simulink model "SModel_VolturnUS"  (R2024b)
settings: Solver=ode4  StartTime=0  StopTime=1000  FixedStep=0.01  MaxStep=0.01  RelTol=1e-3
values from neighbouring files (symbols this model uses):
  simu = simulationClass()    [wecSimInputFile.m]
undefined symbols (not defined in the file or in its folder): body, constraint, mooring, X, Y, Z
libraries: nesl_utility x18, sm_lib x11, WECSim_Lib_Body_Elements x2, WECSim_Lib_Constraints x1, WECSim_Lib_Frames x1, WECSim_Lib_Moorings x1, MOST_Lib x1
settings Model: Creator=massi  LastModifiedBy=akeeste
settings SolverCC: ZeroCrossControl=DisableAll  AlgebraicLoopSolver=TrustRegion  AutoInsertRateTranBlk=on
settings DataIOCC: ReturnWorkspaceOutputs=off
settings OptimizationCC: ReuseModelBlockBuffer=off  SimCompilerOptimization=on
settings DebuggingCC: UnconnectedInputMsg=warning  UnconnectedOutputMsg=warning  UnconnectedLineMsg=warning
settings ModelReferenceCC: EnableRefExpFcnMdlSchedulingChecks=on
settings RTWCC: GPUComputeCapability=3.5
settings ExplorerConfigSet: InternalSimMechanicsExplorerSettings="<ExplorerConfiguration><canonicalview>default</canonicalview><AnimationSetting><BasePlaybackSpeed>1.0</BasePlaybackSpeed><PlaybackSpeedFactor>64.0</PlaybackSpeedFactor></AnimationSetting><TilePanel><TileInfo><Tiles Columns=\"1\" Count=\"1\" Rows=\"1\"><Column Weight=\"1\"/><Row Weight=\"1\"/><Tile Height=\"1\" Width=\"1\" X=\"0\" Y=\"0\"/></Tiles></TileInfo><SceneInfo><SceneViewer><BGColor><R>0.800000011920928955</R><G>1</G><B>1</B></BGColor><Camera><DoPerspective>off</DoPerspective><Position><X>3.83527572012098972e-06</X><Y>-435.132249170182718</Y><Z>-23.2456610583153065</Z></Position><Center><X>3.83527572012098972e-06</X><Y>-1.30964724540660882e-05</Y><Z>-23.2456610583153065</Z></Center><Up><X>0</X><Y>-0</Y><Z>1</Z></Up><ViewLimDist>1</ViewLimDist><YLim>286.086963500976594</YLim><XLim>444.426516742997762</XLim></Camera></SceneViewer></SceneInfo></TilePanel><MechEditorPanel><Cameras/><GfxPanelCameraMap/><VideoCreator><PlaybackSpeedRatio>1.0</PlaybackSpeedRatio><FrameRate>30</FrameRate><VideoFormat>Motion JPEG AVI</VideoFormat><FrameSize>auto</FrameSize></VideoCreator></MechEditorPanel></ExplorerConfiguration>"

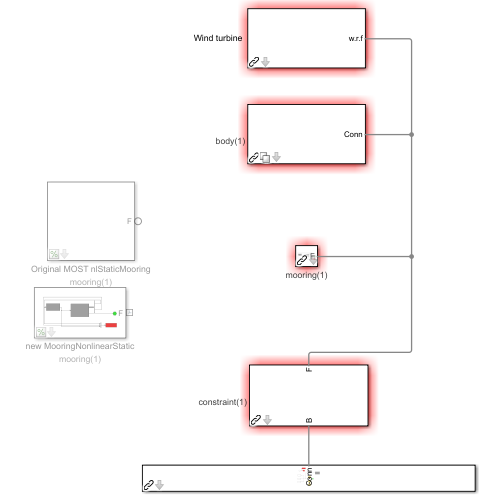
[thumbnail: Simulink's stored preview of the top-level diagram]
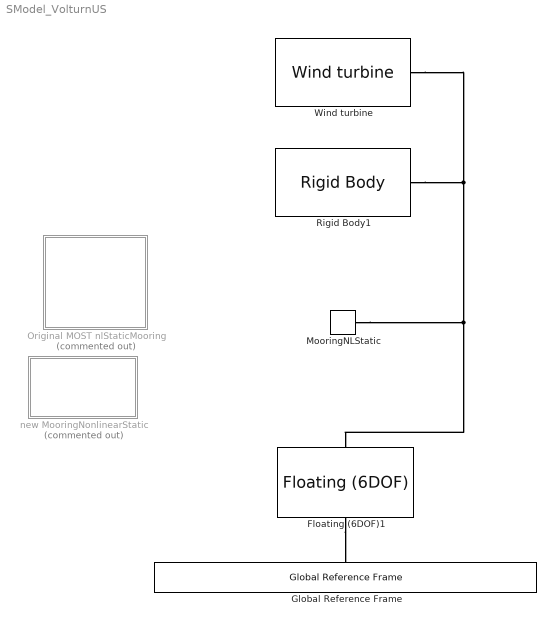
== system SModel_VolturnUS ==
  Floating (6DOF)1 : WECSim_Lib_Constraints/Floating (6DOF)  constraint=constraint(1)
      settings: AttributesFormatString=%<constraint>
  Global Reference Frame : WECSim_Lib_Frames/Global Reference Frame  waves=waves  simu=simu
  MooringNLStatic : WECSim_Lib_Moorings/MooringNLStatic  mooring=mooring(1)  nonlinearStaticData=mooring.nonlinearStaticData
      settings: AttributesFormatString=%<mooring>
  Original MOST nlStaticMooring : Subsystem  Commented=on  mask{mooring=mooring(1), Data_moor=mooring(1).nonlinearStaticData}
      mask prompts: mooring "Mooring Name:"; Data_moor "Mooring Data"
      mask init:
      | if exist('mooring','var')
      |     % toWorkSpace: outputs
      |     h=[gcb '/To Workspace'];
      |     responseName=['mooring' num2str(mooring.number) '_out'];
      |     set_param(h,'VariableName',responseName);
      | end
      settings: AttributesFormatString=%<mooring>
  Rigid Body1 : WECSim_Lib_Body_Elements/Rigid Body  body=body(1)
  Wind turbine : MOST_Lib/Wind turbine  VariantControl=sv_1_IEA15MW  windTurbine=windTurbine  BEMstruct=windTurbine.BEMstruct
      settings: SourceProductName=MOST
  new MooringNonlinearStatic : Subsystem  Commented=on  mask(Mooring Matrix){mooring=mooring(1), nonlinearStaticData=mooring.nonlinearStaticData}
      mask prompts: mooring "Mooring Name:"; nonlinearStaticData "Mooring Data"
      mask help:
      | A mooring body that applies stiffness, damping and pretensions forces to the follower. The response of the mooring body is relative to the global reference frame.
      |
      | The variable name input below must be 'mooring(i)' where i=1,2,...
      | mooring(i) must be defined in the input file with the following fields:
      |
      |     .name (required)
      |             String.
      |             Mooring name. Must comply with Matlab's variable naming rules.
      |     .location (optional)
      |             3x1 vector [x y z] in meters.
      |             Mooring location. Default = [0 0 0]
      |     .initial (optional)
      |             Struct
      |             Contains the initial position, angle and axis of the mooring body.
      |     .initial.displacement (optional)
      |             3x1 vector [x y z] in meters.
      |             Initial linear displacement from the ref position. Default = [0 0 0]
      |             This can can be set directly or with the setInitDisp() method.
      |     .initial.axis (optional)
      |             3x1 vector [x y z]
      |             Initial angular displacement axis. Default = [0 1 0]
      |             This can can be set directly or with the setInitDisp() method.
      |     .initial.angle (optional)
      |             Float.
      |             Initial angular displacement angle about axis in radians. Default = [0 0 0]
      |             This can can be set directly or with the setInitDisp() method.
      |     .matrix (optional)
      |             Struct
      |             Contains the stiffness matrix, damping matrix and pretension of the mooring body.
      |     .matrix.stiffness (optional)
      |             6x6 vector.
      |             Mooring linear spring stiffness. Default = zeros(6)
      |     .matrix.damping (optional)
      |             6x6 vector.
      |             Mooring linear damping coefficient. Default = zeros(6)
      |     .matrix.preTension (optional)
      |             6x1 vector.
      |             Mooring preTension force. Default = [0 0 0 0 0 0]
      mask init:
      | if exist('mooring','var')
      |     % toWorkSpace: outputs
      |     h=[gcb '/To Workspace'];
      |     responseName=['mooring' num2str(mooring.number) '_out'];
      |     set_param(h,'VariableName',responseName);
      | end
      settings: AttributesFormatString=%<mooring>
      mask Help:
      | A mooring body that applies stiffness, damping and pretensions forces to the follower. The response of the mooring body is relative to the global reference frame.
      | 
      | The variable name input below must be 'mooring(i)' where i=1,2,...
      | mooring(i) must be defined in the input file with the following fields:
      | 
      |     .name (required)
      |             String.
      |             Mooring name. Must comply with Matlab's variable naming rules.
      |     .location (optional)
      |             3x1 vector [x y z] in meters.
      |             Mooring location. Default = [0 0 0]
      |     .initial (optional)
      |             Struct
      |             Contains the initial position, angle and axis of the mooring body.
      |     .initial.displacement (optional)
      |             3x1 vector [x y z] in meters.
      |             Initial linear displacement from the ref position. Default = [0 0 0]
      |             This can can be set directly or with the setInitDisp() method.
      |     .initial.axis (optional)
      |             3x1 vector [x y z]
      |             Initial angular displacement axis. Default = [0 1 0]
      |             This can can be set directly or with the setInitDisp() method.
      |     .initial.angle (optional)
      |             Float.
      |             Initial angular displacement angle about axis in radians. Default = [0 0 0]
      |             This can can be set directly or with the setInitDisp() method.
      |     .matrix (optional)
      |             Struct
      |             Contains the stiffness matrix, damping matrix and pretension of the mooring body.
      |     .matrix.stiffness (optional)
      |             6x6 vector.
      |             Mooring linear spring stiffness. Default = zeros(6)
      |     .matrix.damping (optional)
      |             6x6 vector.
      |             Mooring linear damping coefficient. Default = zeros(6)
      |     .matrix.preTension (optional)
      |             6x1 vector.
      |             Mooring preTension force. Default = [0 0 0 0 0 0]
  connections:
  Rigid Body1/RConn1 -- Wind turbine/RConn1 -- MooringNLStatic/LConn1 -- Floating (6DOF)1/RConn1
  Floating (6DOF)1/LConn1 -- Global Reference Frame/RConn1

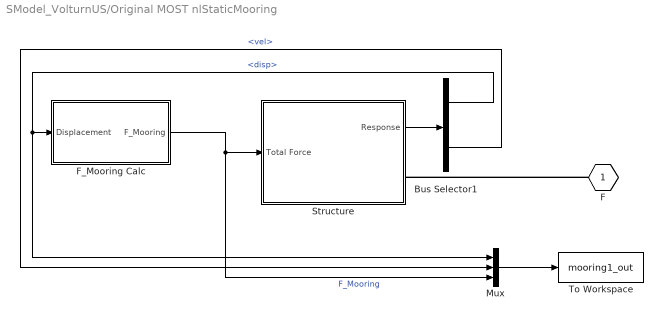
== system SModel_VolturnUS/Original MOST nlStaticMooring ==
  Bus Selector1 : BusSelector  OutputSignals=disp,vel
  F_Mooring Calc : Subsystem
  Mux : Mux  Inputs=3
  Structure : Subsystem
  To Workspace : ToWorkspace  VariableName=mooring1_out  SaveFormat=Structure With Time  SampleTime=simu.dtOut
  F : PMIOPort  Side=Left
  wires:
  Mux/1 -> To Workspace/1
  Bus Selector1/2 -> Mux/2  "<vel>"
  Bus Selector1/1 -> Mux/1, F_Mooring Calc/1(Displacement)  "<disp>"
  F_Mooring Calc/1(F_Mooring) -> Mux/3, Structure/1(Total Force)  "F_Mooring"
  Structure/1(Response) -> Bus Selector1/1
  connections:
  F/RConn1 -- Structure/RConn1

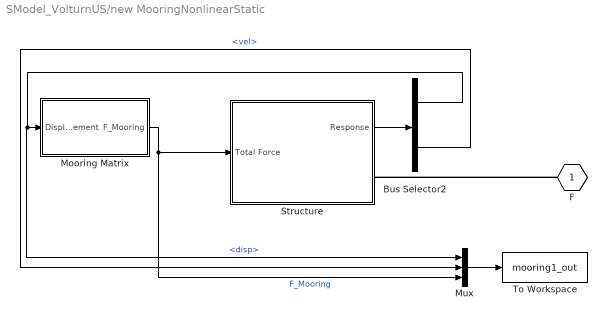
== system SModel_VolturnUS/new MooringNonlinearStatic ==
  Bus Selector2 : BusSelector  OutputSignals=disp,vel
  Mooring Matrix : Subsystem  VariantControl=sv_mooringMatrix
  Mux : Mux  Inputs=3
  Structure : Subsystem
  To Workspace : ToWorkspace  VariableName=mooring1_out  SaveFormat=Structure With Time  SampleTime=simu.dtOut
  F : PMIOPort  Side=Left
  wires:
  Mux/1 -> To Workspace/1
  Bus Selector2/2 -> Mux/2  "<vel>"
  Bus Selector2/1 -> Mooring Matrix/1(Displacement), Mux/1  "<disp>"
  Mooring Matrix/1(F_Mooring) -> Structure/1(Total Force), Mux/3  "F_Mooring"
  Structure/1(Response) -> Bus Selector2/1
  connections:
  F/RConn1 -- Structure/RConn1

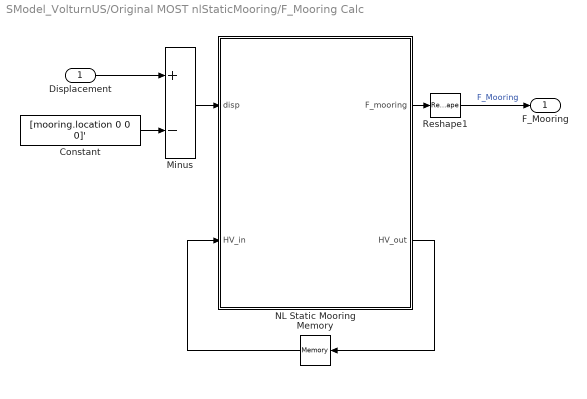
== system SModel_VolturnUS/Original MOST nlStaticMooring/F_Mooring Calc ==
  Displacement : Inport
  Constant : Constant  Value=[mooring.location 0 0 0]'
  Memory : Memory  InitialCondition=Data_moor.HV0
  Minus : Sum  Inputs=+-
  NL Static Mooring : MATLAB Function  TreatAsAtomicUnit=on
  Reshape1 : Reshape
  F_Mooring : Outport
  wires:
  NL Static Mooring/1(F_mooring) -> Reshape1/1
  Displacement/1 -> Minus/1
  Constant/1 -> Minus/2
  Minus/1 -> NL Static Mooring/1(disp)
  Memory/1 -> NL Static Mooring/2(HV_in)
  NL Static Mooring/2(HV_out) -> Memory/1
  Reshape1/1 -> F_Mooring/1  "F_Mooring"

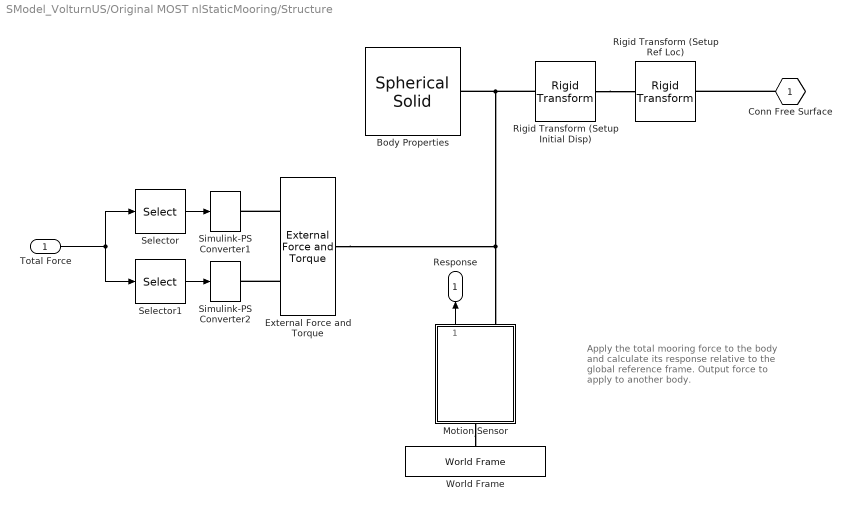
== system SModel_VolturnUS/Original MOST nlStaticMooring/Structure ==
  note: Apply the total mooring force to the body and calculate its response relative to the global reference frame.
      |
      | Output force to apply to another body.
  Total Force : Inport
  Body Properties : sm_lib/Body Elements/Spherical Solid  GraphicAmbientColor=[0.15 0.15 0.15 1.0]  BasedOnType=Density  CenterOfMass=[0 0 0]  CenterOfMassUnits=m  GraphicDiffuseColor=[0.4 0.4 0.4]  Density=1000  DensityUnits=kg/(m^3)  DoExposeReferenceFrame=on  GraphicEmissiveColor=[0.0 0.0 0.0 1.0]  ExportEntireGeometry=off  SerializedExposedGeometries=<ExposedGeometries/>  SerializedFrames=<Frames/>  MarkerShape=Sphere  MarkerSize=10  GraphicType=None  InertiaType=Custom  Mass=0  MassUnits=kg  MomentsOfInertia=[0 0 0]  MomentsOfInertiaUnits=kg*m^2  GraphicOpacity=1  ProductsOfInertia=[0 0 0]  ProductsOfInertiaUnits=kg*m^2  GraphicShininess=75  GraphicSpecularColor=[0.5 0.5 0.5 1.0]  SphereRadius=5  SphereRadiusUnits=m  GraphicVisPropType=SimpleVisualProperties
  External Force and Torque : sm_lib/Forces and Torques/External Force and Torque  ForceResolutionFrame=World  EnableForceX=off  EnableForceY=off  EnableForceZ=off  EnableForce=on  TorqueResolutionFrame=World  EnableTorqueX=off  EnableTorqueY=off  EnableTorqueZ=off  EnableTorque=on
  Motion Sensor : Subsystem
  Rigid Transform (Setup Initial Disp) : sm_lib/Frames and Transforms/Rigid Transform  TranslationMethod=Cartesian  TranslationStandardOffset=0  TranslationStandardOffsetUnits=m  TranslationStandardAxis=+Z  TranslationCartesianOffset=mooring.initial.displacement  TranslationCartesianOffsetUnits=m  TranslationROffset=0  TranslationROffsetUnits=m  TranslationZOffset=0  TranslationZOffsetUnits=m  TranslationThetaOffset=0  TranslationThetaOffsetUnits=deg  RotationMethod=ArbitraryAxis  RotationAngleUnits=rad  RotationStandardAxis=+Y  RotationAngle=mooring.initial.angle  RotationArbitraryAxis=mooring.initial.axis  FollAlignAxisA=+X  BaseAlignAxisA=+Y  FollAlignAxisB=+Y  BaseAlignAxisB=+Z  RotationSequenceAxes=FollowerAxes  RotationSequence=XYX  RotationSequenceAngles=[0 0 0]  RotationSequenceAnglesUnits=deg  RotationMatrix=[1 0 0; 0 1 0; 0 0 1]  Quaternion=[1 0 0 0]
  Rigid Transform (Setup Ref Loc) : sm_lib/Frames and Transforms/Rigid Transform  TranslationMethod=Cartesian  TranslationStandardOffset=0  TranslationStandardOffsetUnits=m  TranslationStandardAxis=+Z  TranslationCartesianOffset=mooring.location  TranslationCartesianOffsetUnits=m  TranslationROffset=0  TranslationROffsetUnits=m  TranslationZOffset=0  TranslationZOffsetUnits=m  TranslationThetaOffset=0  TranslationThetaOffsetUnits=deg  RotationMethod=None  RotationAngleUnits=rad  RotationStandardAxis=+Y  RotationAngle=0.05  RotationArbitraryAxis=[0.57735026918962584 0.57735026918962584 0.57735026918962584]  FollAlignAxisA=+X  BaseAlignAxisA=+Y  FollAlignAxisB=+Y  BaseAlignAxisB=+Z  RotationSequenceAxes=FollowerAxes  RotationSequence=XYX  RotationSequenceAngles=[0 0 0]  RotationSequenceAnglesUnits=deg  RotationMatrix=[1 0 0; 0 1 0; 0 0 1]  Quaternion=[1 0 0 0]
  Selector : Selector  InputPortWidth=6  IndexOptions=Index vector (dialog)  Indices=[1:3]  OutputSizes=1
  Selector1 : Selector  InputPortWidth=6  IndexOptions=Index vector (dialog)  Indices=[4:6]  OutputSizes=1
  Simulink-PS Converter1 : nesl_utility/Simulink-PS Converter  PhysicalDomain=network_engine_domain  SubClassName=ps_input  LeftPortType=input  RightPortType=output  PseudoPeriodic=off  Frequencies=[]  NoiseDistribution=none  NoiseParameters=[]  Unit=1  AffineConversion=off  FilteringAndDerivatives=zero  SimscapeFilterOrder=1  InputFilterTimeConstant=0.001  UdotUserProvided=1
  Simulink-PS Converter2 : nesl_utility/Simulink-PS Converter  PhysicalDomain=network_engine_domain  SubClassName=ps_input  LeftPortType=input  RightPortType=output  PseudoPeriodic=off  Frequencies=[]  NoiseDistribution=none  NoiseParameters=[]  Unit=1  AffineConversion=off  FilteringAndDerivatives=zero  SimscapeFilterOrder=1  InputFilterTimeConstant=0.001  UdotUserProvided=1
  World Frame : sm_lib/Frames and Transforms/World Frame
  Conn Free Surface : PMIOPort  Side=Right
  Response : Outport
  wires:
  Motion Sensor/1(Response) -> Response/1
  Selector1/1 -> Simulink-PS Converter2/1
  Selector/1 -> Simulink-PS Converter1/1
  Total Force/1 -> Selector/1, Selector1/1
  connections:
  Motion Sensor/LConn1 -- World Frame/RConn1
  Rigid Transform (Setup Initial Disp)/LConn1 -- Rigid Transform (Setup Ref Loc)/RConn1
  Conn Free Surface/RConn1 -- Rigid Transform (Setup Ref Loc)/LConn1
  Body Properties/RConn1 -- Rigid Transform (Setup Initial Disp)/RConn1 -- External Force and Torque/RConn1 -- Motion Sensor/RConn1
  External Force and Torque/LConn2 -- Simulink-PS Converter2/RConn1
  External Force and Torque/LConn1 -- Simulink-PS Converter1/RConn1

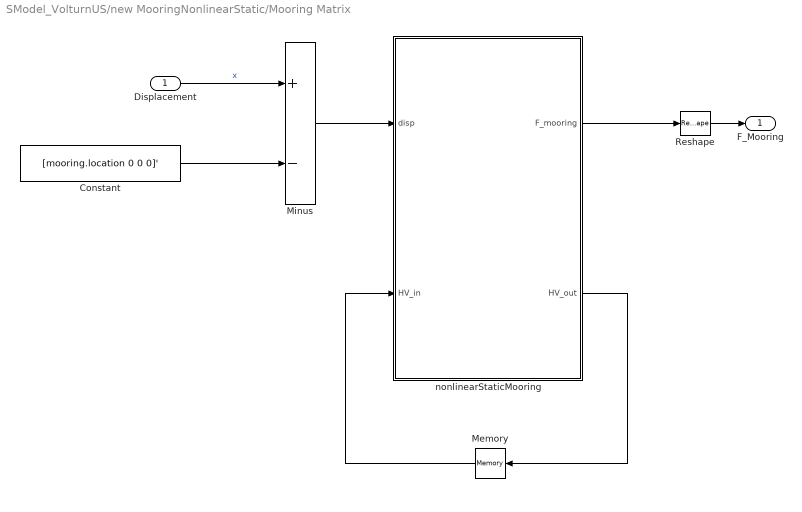
== system SModel_VolturnUS/new MooringNonlinearStatic/Mooring Matrix ==
  Displacement : Inport
  Constant : Constant  Value=[mooring.location 0 0 0]'
  Memory : Memory  InitialCondition=nonlinearStaticData.HV0
  Minus : Sum  Inputs=+-
  Reshape : Reshape
  nonlinearStaticMooring : MATLAB Function  TreatAsAtomicUnit=on
  F_Mooring : Outport
  wires:
  Reshape/1 -> F_Mooring/1
  Displacement/1 -> Minus/1  "x"
  Constant/1 -> Minus/2
  nonlinearStaticMooring/1(F_mooring) -> Reshape/1
  nonlinearStaticMooring/2(HV_out) -> Memory/1
  Memory/1 -> nonlinearStaticMooring/2(HV_in)
  Minus/1 -> nonlinearStaticMooring/1(disp)

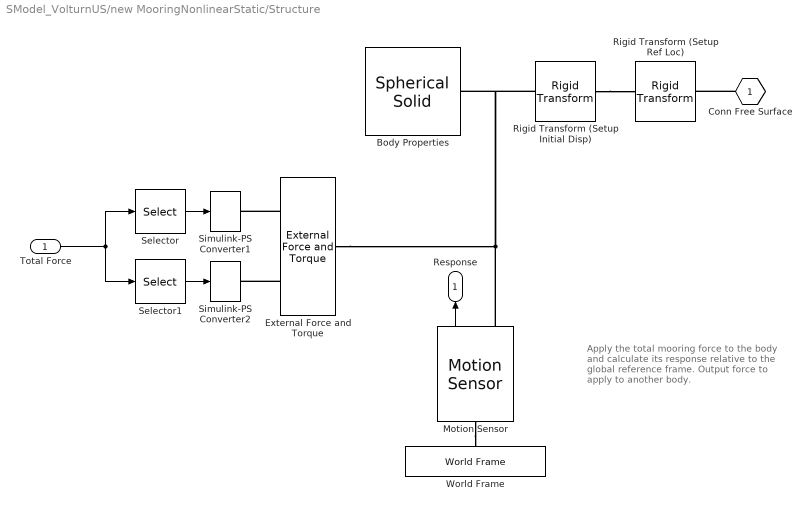
== system SModel_VolturnUS/new MooringNonlinearStatic/Structure ==
  note: Apply the total mooring force to the body and calculate its response relative to the global reference frame.
      |
      | Output force to apply to another body.
  Total Force : Inport
  Body Properties : sm_lib/Body Elements/Spherical Solid  SphereRadius=1  SphereRadiusUnits=m  ExportEntireGeometry=off  InertiaType=Custom  BasedOnType=Density  Density=1000  DensityUnits=kg/(m^3)  Mass=0  MassUnits=kg  CenterOfMass=[0 0 0]  CenterOfMassUnits=m  MomentsOfInertia=[0 0 0]  MomentsOfInertiaUnits=kg*m^2  ProductsOfInertia=[0 0 0]  ProductsOfInertiaUnits=kg*m^2  GraphicType=None  MarkerShape=Sphere  MarkerSize=10  GraphicVisPropType=SimpleVisualProperties  GraphicDiffuseColor=[0 1 0]  GraphicOpacity=1  GraphicSpecularColor=[0.5 0.5 0.5 1.0]  GraphicAmbientColor=[0.15 0.15 0.15 1.0]  GraphicEmissiveColor=[0.0 0.0 0.0 1.0]  GraphicShininess=75  DoExposeReferenceFrame=on  SerializedFrames=<Frames/>
  External Force and Torque : sm_lib/Forces and Torques/External Force and Torque  EnableForceX=off  EnableForceY=off  EnableForceZ=off  EnableForce=on  ForceResolutionFrame=World  EnableTorqueX=off  EnableTorqueY=off  EnableTorqueZ=off  EnableTorque=on  TorqueResolutionFrame=World
  Motion Sensor : WECSim_Lib_Body_Elements/Rigid Body/Hydrodynamic Body/Structure/Motion Sensor  SystemSampleTime=-1  VariantActivationTime=update diagram  AllowFlexibleInterface=on  Latency=0  AutoFrameSizeCalculation=off
  Rigid Transform (Setup Initial Disp) : sm_lib/Frames and Transforms/Rigid Transform  RotationMethod=ArbitraryAxis  FollAlignAxisA=+X  BaseAlignAxisA=+Y  FollAlignAxisB=+Y  BaseAlignAxisB=+Z  RotationStandardAxis=+Y  RotationAngle=mooring.initial.angle  RotationAngleUnits=rad  RotationArbitraryAxis=mooring.initial.axis  RotationSequenceAxes=FollowerAxes  RotationSequence=XYX  RotationSequenceAngles=[0 0 0]  RotationSequenceAnglesUnits=deg  RotationMatrix=[1 0 0; 0 1 0; 0 0 1]  Quaternion=[1 0 0 0]  TranslationMethod=Cartesian  TranslationCartesianOffset=mooring.initial.displacement  TranslationCartesianOffsetUnits=m  TranslationStandardAxis=+Z  TranslationStandardOffset=0  TranslationStandardOffsetUnits=m  TranslationROffset=0  TranslationROffsetUnits=m  TranslationThetaOffset=0  TranslationThetaOffsetUnits=deg  TranslationZOffset=0  TranslationZOffsetUnits=m
  Rigid Transform (Setup Ref Loc) : sm_lib/Frames and Transforms/Rigid Transform  RotationMethod=None  FollAlignAxisA=+X  BaseAlignAxisA=+Y  FollAlignAxisB=+Y  BaseAlignAxisB=+Z  RotationStandardAxis=+Y  RotationAngle=0.05  RotationAngleUnits=rad  RotationArbitraryAxis=[0.57735026918962584 0.57735026918962584 0.57735026918962584]  RotationSequenceAxes=FollowerAxes  RotationSequence=XYX  RotationSequenceAngles=[0 0 0]  RotationSequenceAnglesUnits=deg  RotationMatrix=[1 0 0; 0 1 0; 0 0 1]  Quaternion=[1 0 0 0]  TranslationMethod=Cartesian  TranslationCartesianOffset=mooring.location  TranslationCartesianOffsetUnits=m  TranslationStandardAxis=+Z  TranslationStandardOffset=0  TranslationStandardOffsetUnits=m  TranslationROffset=0  TranslationROffsetUnits=m  TranslationThetaOffset=0  TranslationThetaOffsetUnits=deg  TranslationZOffset=0  TranslationZOffsetUnits=m
  Selector : Selector  InputPortWidth=6  IndexOptions=Index vector (dialog)  Indices=[1:3]  OutputSizes=1
  Selector1 : Selector  InputPortWidth=6  IndexOptions=Index vector (dialog)  Indices=[4:6]  OutputSizes=1
  Simulink-PS Converter1 : nesl_utility/Simulink-PS Converter  PhysicalDomain=network_engine_domain  SubClassName=ps_input  LeftPortType=input  RightPortType=output  PseudoPeriodic=off  Frequencies=[]  NoiseDistribution=none  NoiseParameters=[]  Unit=1  AffineConversion=off  FilteringAndDerivatives=zero  SimscapeFilterOrder=1  InputFilterTimeConstant=0.001  UdotUserProvided=1
  Simulink-PS Converter2 : nesl_utility/Simulink-PS Converter  PhysicalDomain=network_engine_domain  SubClassName=ps_input  LeftPortType=input  RightPortType=output  PseudoPeriodic=off  Frequencies=[]  NoiseDistribution=none  NoiseParameters=[]  Unit=1  AffineConversion=off  FilteringAndDerivatives=zero  SimscapeFilterOrder=1  InputFilterTimeConstant=0.001  UdotUserProvided=1
  World Frame : sm_lib/Frames and Transforms/World Frame
  Conn Free Surface : PMIOPort  Side=Right
  Response : Outport
  wires:
  Motion Sensor/1 -> Response/1
  Selector1/1 -> Simulink-PS Converter2/1
  Selector/1 -> Simulink-PS Converter1/1
  Total Force/1 -> Selector/1, Selector1/1
  connections:
  Motion Sensor/LConn1 -- World Frame/RConn1
  Rigid Transform (Setup Initial Disp)/LConn1 -- Rigid Transform (Setup Ref Loc)/RConn1
  Conn Free Surface/RConn1 -- Rigid Transform (Setup Ref Loc)/LConn1
  External Force and Torque/RConn1 -- Motion Sensor/RConn1 -- Body Properties/RConn1 -- Rigid Transform (Setup Initial Disp)/RConn1
  External Force and Torque/LConn2 -- Simulink-PS Converter2/RConn1
  External Force and Torque/LConn1 -- Simulink-PS Converter1/RConn1

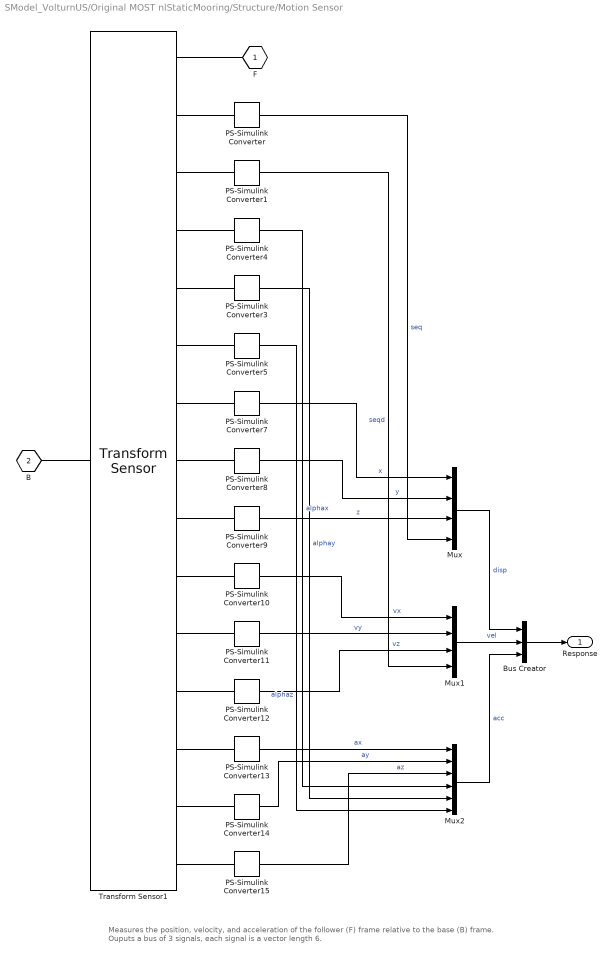
== system SModel_VolturnUS/Original MOST nlStaticMooring/Structure/Motion Sensor ==
  note: Measures the position, velocity, and acceleration of the follower (F) frame relative to the base (B) frame.
      | Ouputs a bus of 3 signals, each signal is a vector length 6.
  Bus Creator : BusCreator  Inputs=3
  Mux : Mux
  Mux1 : Mux
  Mux2 : Mux  Inputs=6
  PS-Simulink Converter{,1,3..5,7..15} (14 alike) : nesl_utility/PS-Simulink Converter  PhysicalDomain=network_engine_domain  SubClassName=ps_output  LeftPortType=input  RightPortType=output  PseudoPeriodic=off  Frequencies=[]  VectorFormat=1-D array  Unit=1  AffineConversion=off
  Transform Sensor1 : sm_lib/Frames and Transforms/Transform Sensor  MeasurementFrame=World  RotationSequence=XYZ  SenseAngle=off  SenseAxis=off  SenseQ=off  SenseR=off  SenseRotationSequence=on  SenseOmegaX=off  SenseOmegaY=off  SenseOmegaZ=off  SenseOmega=off  SenseQDot=off  SenseRDot=off  SenseRotationSequenceDot=on  SenseAlphaX=on  SenseAlphaY=on  SenseAlphaZ=on  SenseAlpha=off  SenseQDDot=off  SenseRDDot=off  SenseX=on  SenseY=on  SenseZ=on  SenseXYZ=off  SenseRad=off  SenseAzim=off  SenseDist=off  SenseInc=off  SenseXDot=on  SenseYDot=on  SenseZDot=on  SenseXYZDot=off  SenseRadDot=off  SenseAzimDot=off  SenseDistDot=off  SenseIncDot=off  SenseXDDot=on  SenseYDDot=on  SenseZDDot=on  SenseXYZDDot=off  SenseRadDDot=off  SenseAzimDDot=off  SenseDistDDot=off  SenseIncDDot=off
  F : PMIOPort  Side=Right
  B : PMIOPort  Port=2  Side=Left
  Response : Outport
  wires:
  PS-Simulink Converter9/1 -> Mux/3  "z"
  PS-Simulink Converter15/1 -> Mux2/3  "az"
  PS-Simulink Converter5/1 -> Mux2/6  "alphaz"
  PS-Simulink Converter12/1 -> Mux1/3  "vz"
  PS-Simulink Converter8/1 -> Mux/2  "y"
  PS-Simulink Converter3/1 -> Mux2/5  "alphay"
  PS-Simulink Converter10/1 -> Mux1/1  "vx"
  PS-Simulink Converter/1 -> Mux/4  "seq"
  PS-Simulink Converter1/1 -> Mux1/4  "seqd"
  PS-Simulink Converter7/1 -> Mux/1  "x"
  PS-Simulink Converter4/1 -> Mux2/4  "alphax"
  Mux1/1 -> Bus Creator/2  "vel"
  PS-Simulink Converter14/1 -> Mux2/2  "ay"
  Bus Creator/1 -> Response/1
  Mux/1 -> Bus Creator/1  "disp"
  Mux2/1 -> Bus Creator/3  "acc"
  PS-Simulink Converter13/1 -> Mux2/1  "ax"
  PS-Simulink Converter11/1 -> Mux1/2  "vy"
  connections:
  Transform Sensor1/RConn1 -- F/RConn1
  Transform Sensor1/LConn1 -- B/RConn1
  Transform Sensor1/RConn5 -- PS-Simulink Converter3/LConn1
  Transform Sensor1/RConn2 -- PS-Simulink Converter/LConn1
  PS-Simulink Converter4/LConn1 -- Transform Sensor1/RConn4
  Transform Sensor1/RConn7 -- PS-Simulink Converter7/LConn1
  PS-Simulink Converter8/LConn1 -- Transform Sensor1/RConn8
  PS-Simulink Converter1/LConn1 -- Transform Sensor1/RConn3
  PS-Simulink Converter15/LConn1 -- Transform Sensor1/RConn15
  Transform Sensor1/RConn13 -- PS-Simulink Converter13/LConn1
  PS-Simulink Converter11/LConn1 -- Transform Sensor1/RConn11
  Transform Sensor1/RConn14 -- PS-Simulink Converter14/LConn1
  Transform Sensor1/RConn6 -- PS-Simulink Converter5/LConn1
  Transform Sensor1/RConn9 -- PS-Simulink Converter9/LConn1
  PS-Simulink Converter10/LConn1 -- Transform Sensor1/RConn10
  PS-Simulink Converter12/LConn1 -- Transform Sensor1/RConn12

== matlab function SModel_VolturnUS/Original MOST nlStaticMooring/F_Mooring Calc/NL Static Mooring ==
  data: disp input size=[6 1]; F_mooring output size=[6 1]; HV_in input double size=size(Data_moor.HV0); Data_moor parameter; HV_out output size=size(Data_moor.HV0)
function [F_mooring,HV_out] = NL_Static_Mooring(disp,HV_in, Data_moor)

F_mooring=zeros(6,1);
HV_out=zeros(Data_moor.nLines,2);
RMat=Rzyx(disp(6),disp(5),disp(4));

for m=1:Data_moor.nLines

    FairleadNotrasl =RMat*Data_moor.nodes(:,2*m-1);
    DX= Data_moor.nodes(:,2*m)-...                          % Anchor
        (FairleadNotrasl+[disp(1);disp(2);disp(3)]);        % Fairlead

    h = abs(DX(3));
    r = norm(DX(1:2));

    [HV_out(m,:)]=fminsearch(@(HV)Calc_HV(HV,h,r,Data_moor),HV_in(m,:),Data_moor.fminsearch_options);

    alpha=atan(DX(2)/DX(1))+pi*(DX(1)<0);
    F=[HV_out(m,1).*[cos(alpha);sin(alpha)];-HV_out(m,2)];
    F_mooring = F_mooring + [F;
        cross(FairleadNotrasl,F)];

end


end


function err = Calc_HV(HV,h,r,Data_moor)

% Calculate the length of the bottom segment of the line
LB=Data_moor.L-HV(2)/Data_moor.w;

if LB > 0  % If the line touchs the seabed
     
    g=LB-HV(1)/Data_moor.CB/Data_moor.w;
    lambda=double(g>0)*g;
       
    x=LB+HV(1)/Data_moor.w*asinh(Data_moor.w*(Data_moor.L-LB)/HV(1))+HV(1)*Data_moor.L/Data_moor.EA+Data_moor.CB*Data_moor.w/2/Data_moor.EA*(g*lambda-LB^2);
    z=HV(1)/Data_moor.w*((sqrt(1+(Data_moor.w*(Data_moor.L-LB)/HV(1)).^2))-1)+Data_moor.w*(Data_moor.L-LB).^2/2/Data_moor.EA;
      
else      % If the line does not touch the seabed
    Va=HV(2)-Data_moor.w*Data_moor.L;
    x = HV(1)/Data_moor.w * (asinh((Va+Data_moor.w*Data_moor.L)/HV(1)) - asinh((Va)/HV(1) )) + HV(1)*Data_moor.L/Data_moor.EA;
    z = HV(1)/Data_moor.w * (sqrt(1+((Va+Data_moor.w*Data_moor.L)/HV(1)).^2) - sqrt(1+(Va/HV(1))^2)) + (Va*Data_moor.L+Data_moor.w*Data_moor.L.^2/2)/Data_moor.EA;
end


err=sqrt((x-r)^2+(z-h)^2);

end


function Rzyx=Rzyx(rz,ry,rx)
  
  Rzyx=[cos(ry)*cos(rz)     sin(rx)*sin(ry)*cos(rz)-cos(rx)*sin(rz)         cos(rx)*sin(ry)*cos(rz)+sin(rx)*sin(rz);

        cos(ry)*sin(rz)     sin(rx)*sin(ry)*sin(rz)+cos(rx)*cos(rz)         cos(rx)*sin(ry)*sin(rz)-sin(rx)*cos(rz);

           -sin(ry)                     sin(rx)*cos(ry)                                  cos(rx)*cos(ry)             ];
end

== matlab function SModel_VolturnUS/new MooringNonlinearStatic/Mooring Matrix/nonlinearStaticMooring ==
  data: disp input size=[6 1]; F_mooring output size=[6 1]; HV_in input size=size(nonlinearStaticData.HV0); HV_out output size=size(nonlinearStaticData.HV0); nonlinearStaticData parameter
function [F_mooring, HV_out] = nlsMooring(disp, HV_in, nonlinearStaticData)

F_mooring = zeros(6, 1);
HV_out = zeros(nonlinearStaticData.nLines, 2);
[F_mooring, HV_out] = nonLinearStaticMooring(disp, HV_in, nonlinearStaticData);

end
